simulink model "rangeSensorProc"  (R2018a)
settings: Solver=FixedStepDiscrete  StartTime=0.0  StopTime=10.0  FixedStep=0.01  RelTol=1e-3
PreLoadFcn:
  | tFilter = 0.01;
  | tFusion = 0.05;
  | 
  | sensData = dlmread('rangeSensorData.txt');
settings Model: Creator=scastro  LastModifiedBy=scastro
settings DataIOCC: ExternalInput=sensData  LoadExternalInput=on  SaveOutput=off  SaveTime=off
settings OptimizationCC: DefaultParameterBehavior=Inlined  EnhancedBackFolding=on  PassReuseOutputArgsAs=Individual arguments  OptimizeBlockOrder=speed  DifferentSizesBufferReuse=on  OptimizationCustomize=off
settings DebuggingCC: ParameterTunabilityLossMsg=error  LibraryContextMissingDiagnostic=warning
settings SFSimCC: SimUseLocalCustomCode=on  MATLABDynamicMemAlloc=off
settings RTWCC: SystemTargetFile=ert.tlc  TemplateMakefile=ert_default_tmf  GenerateReport=on  RTWUseLocalCustomCode=on  IncludeHyperlinkInReport=on  LaunchReport=on  GenerateTraceInfo=on  GenerateTraceReport=on  GenerateTraceReportSl=on  GenerateTraceReportSf=on  GenerateTraceReportEml=on
settings CodeAppCC: ForceParamTrailComments=on  IgnoreCustomStorageClasses=off  OperatorAnnotations=on  SimulinkDataObjDesc=on  SFDataObjDesc=on  InsertBlockDesc=on
settings ERTTargetCC: TargetLangStandard=C99 (ISO)  GenerateSampleERTMain=on  InlinedParameterPlacement=NonHierarchical  ERTCustomFileTemplate=example_file_process.tlc

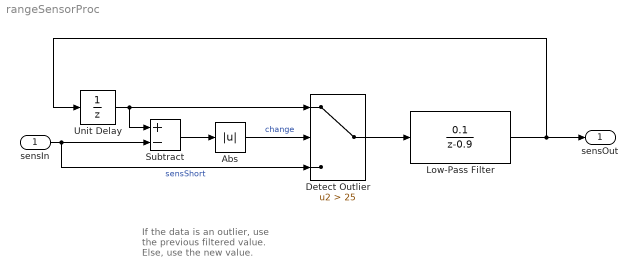
== system rangeSensorProc ==
  note: If the data is an outlier, use the previous filtered value.
      | Else, use the new value.
  sensIn : Inport  OutDataTypeStr=double  PortDimensions=1  SampleTime=[0.01,0]
  Abs : Abs
  Detect Outlier : Switch  Criteria=u2 > Threshold  Threshold=25
  Low-Pass Filter : DiscreteTransferFcn  Numerator=[0.1]  Denominator=[1 -0.9]  SampleTime=tFilter
  Subtract : Sum  Inputs=+-
  Unit Delay : UnitDelay  SampleTime=-1
  sensOut : Outport  OutDataTypeStr=double  PortDimensions=1  SampleTime=[0.01,0]
  wires:
  sensIn/1 -> Detect Outlier/3, Subtract/2  "sensShort"
  Detect Outlier/1 -> Low-Pass Filter/1
  Low-Pass Filter/1 -> Unit Delay/1, sensOut/1
  Unit Delay/1 -> Detect Outlier/1, Subtract/1
  Abs/1 -> Detect Outlier/2  "change"
  Subtract/1 -> Abs/1
